simulink model "Model1"  (R2016a)
settings: Solver=VariableStepAuto  StartTime=0.0  StopTime=10.0  RelTol=1e-3
values from neighbouring files (symbols this model uses):
  B = 0.18e-3    (= 0.00018)    [MotorParameters.m]
  J_l = 1800e-7    (= 0.00018)    [MotorParameters.m]
  J_m = 2118e-7    (= 0.0002118)    [MotorParameters.m]
  Ke = 0.08    [MotorParameters.m]
  Kstif = 7.5    [MotorParameters.m]
  L = 0.9e-3    (= 0.0009)    [MotorParameters.m]
  N1 = 2    [MotorParameters.m]
  N2 = 1    [MotorParameters.m]
  R = 0.43    [MotorParameters.m]
  Tload = 0.75    [MotorParameters.m]
  Vin = 24    [MotorParameters.m]
settings Model: Creator=mrsmash  LastModifiedBy=mrsmash

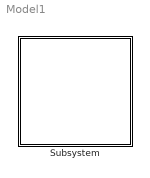
== system Model1 ==
  Subsystem : Subsystem

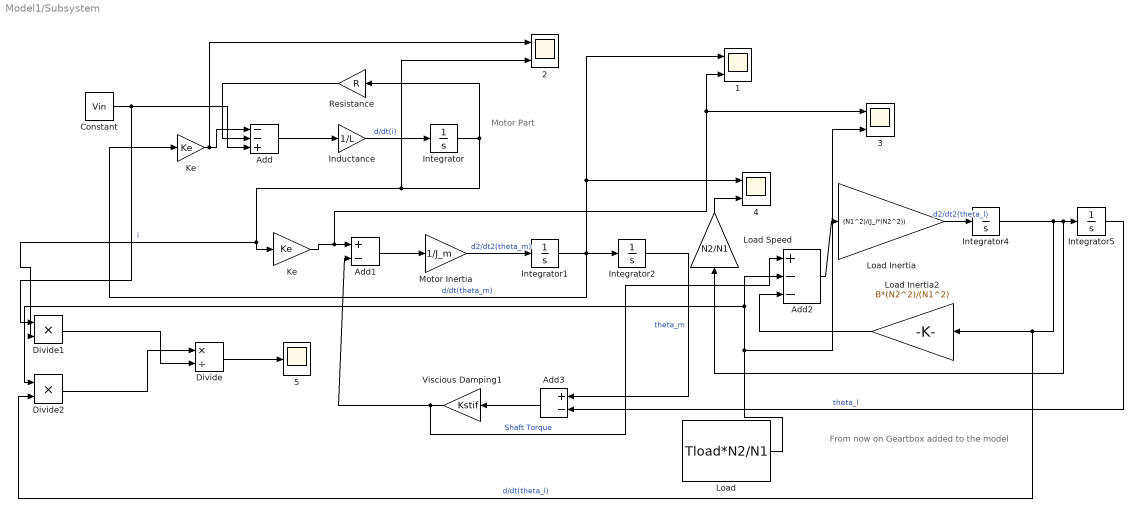
== system Model1/Subsystem ==
  note: From now on Geartbox added to the model
  note: Motor Part
  {1..4} (4 alike) : Scope  NumInputPorts=2
  5 : Scope
  Add : Sum  Inputs=--+
  Add1 : Sum  Inputs=+-
  Add2 : Sum  Inputs=+--
  Add3 : Sum  Inputs=+-
  Constant : Constant  Value=Vin
  Divide : Product  Inputs=*/
  Divide1 : Product  Inputs=**
  Divide2 : Product  Inputs=**
  "Inductance " : Gain  Gain=1/L
  Integrator{,1..2,4..5} (5 alike) : Integrator
  Ke : Gain  Gain=Ke
  "Ke " : Gain  Gain=Ke
  Load : Constant  Value=Tload*N2/N1  SampleTime=-1
  Load Inertia : Gain  Gain=(N1^2)/(J_l*(N2^2))
  Load Inertia2 : Gain  Gain=B*(N2^2)/(N1^2)
  Load Speed : Gain  Gain=N2/N1
  Motor Inertia : Gain  Gain=1/J_m
  Resistance : Gain  Gain=R
  Viscious Damping1 : Gain  Gain=Kstif
  wires:
  Integrator1/1 -> Ke/1, 1/1, 4/1, Integrator2/1  "d/dt(theta_m)"
  Integrator/1 -> Resistance/1, 2/2, Divide1/2, "Ke "/1  "i"
  Add1/1 -> Motor Inertia/1
  Load/1 -> 3/2, Divide2/1, Add2/2
  Integrator2/1 -> Add3/1  "theta_m"
  "Inductance "/1 -> Integrator/1  "d/dt(i)"
  Add/1 -> "Inductance "/1
  Motor Inertia/1 -> Integrator1/1  "d2/dt2(theta_m)"
  "Ke "/1 -> 3/1, 1/2, Add1/1
  Constant/1 -> Divide1/1, Add/3
  Ke/1 -> 2/1, Add/1
  Resistance/1 -> Add/2
  Integrator4/1 -> Divide2/2, Load Inertia2/1, Load Speed/1, Integrator5/1  "d/dt(theta_l)"
  Viscious Damping1/1 -> Add2/1, Add1/2  "Shaft Torque"
  Load Inertia/1 -> Integrator4/1  "d2/dt2(theta_l)"
  Integrator5/1 -> Add3/2  "theta_l"
  Add3/1 -> Viscious Damping1/1
  Load Inertia2/1 -> Add2/3
  Add2/1 -> Load Inertia/1
  Load Speed/1 -> 4/2
  Divide/1 -> 5/1
  Divide2/1 -> Divide/1
  Divide1/1 -> Divide/2
